simulink model "problem1"  (R2020b)
settings: Solver=VariableStepAuto  StartTime=0.0  StopTime=50.0  RelTol=1e-3
model workspace (MAT data in the model file):
  K1 = 50
  K12 = 200
  M1 = 100
  M2 = 60
  b = 50
settings Model: Creator=Admin  LastModifiedBy=Admin

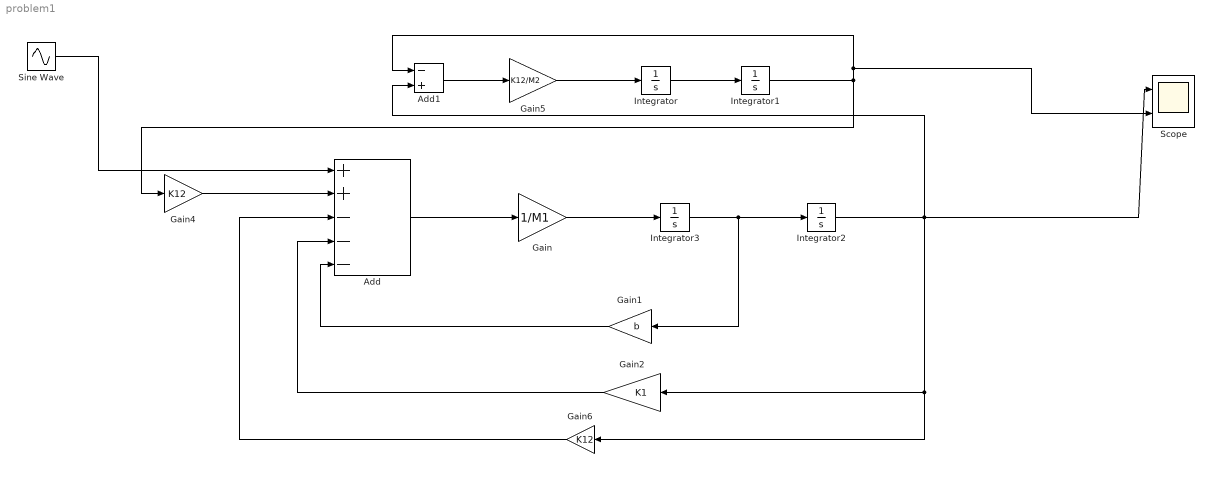
== system problem1 ==
  Add : Sum  Inputs=++---
  Add1 : Sum  Inputs=-+
  Gain : Gain  Gain=1/M1
  Gain1 : Gain  Gain=b
  Gain2 : Gain  Gain=K1
  Gain4 : Gain  Gain=K12
  Gain5 : Gain  Gain=K12/M2
  Gain6 : Gain  Gain=K12
  Integrator{,1..3} (4 alike) : Integrator
  Scope : Scope  NumInputPorts=2
  Sine Wave : Sin  Frequency=10  SampleTime=0
  wires:
  Gain4/1 -> Add/2
  Add1/1 -> Gain5/1
  Gain5/1 -> Integrator/1
  Integrator/1 -> Integrator1/1
  Integrator1/1 -> Scope/2, Add1/1, Gain4/1
  Add/1 -> Gain/1
  Gain/1 -> Integrator3/1
  Integrator3/1 -> Gain1/1, Integrator2/1
  Gain1/1 -> Add/5
  Gain2/1 -> Add/4
  Integrator2/1 -> Add1/2, Scope/1, Gain2/1, Gain6/1
  Gain6/1 -> Add/3
  Sine Wave/1 -> Add/1
